simulink model "formula"  (R2019a)
settings: Solver=VariableStepAuto  StartTime=0.0  StopTime=20  RelTol=1e-3
values from neighbouring files (symbols this model uses):
  a0 = 1.3    [mf.mat]    (also in model_2r.m; model_Fy.m)
  a1 = -0.0274    [mf.mat]    (also in model_2r.m; model_Fy.m)
  a10 = 0.015    [mf.mat]    (also in model_2r.m; model_Fy.m)
  a11 = 0.00849    [mf.mat]    (also in model_2r.m = 0.0849; model_Fy.m)
  a12 = -0.0103    [mf.mat]    (also in model_2r.m; model_Fy.m)
  a13 = 0.0395    [mf.mat]    (also in model_2r.m; model_Fy.m)
  a2 = 1.05    [mf.mat]    (also in model_2r.m; model_Fy.m)
  a3 = 1.18    [mf.mat]    (also in model_2r.m; model_Fy.m)
  a4 = 7.69    [mf.mat]    (also in model_2r.m; model_Fy.m)
  a5 = 0.009    [mf.mat]    (also in model_2r.m; model_Fy.m)
  a6 = -0.257    [mf.mat]    (also in model_2r.m; model_Fy.m)
  a7 = 0.224    [mf.mat]    (also in model_2r.m; model_Fy.m)
  a8 = 0.025    [mf.mat]    (also in model_2r.m; model_Fy.m)
  a9 = 0.01    [mf.mat]    (also in model_2r.m; model_Fy.m)
  Iz = 1500    [mf.mat]    (also in model_2r.m)
  lf = 1.4    [mf.mat]    (also in model_2r.m = 1.2)
  lr = 1.2    [mf.mat]    (also in model_2r.m = 1.4)
  m = 1200    [mf.mat]    (also in model_2r.m)
  V = v/3.6    (= 27.7777777778)    [model_2r.m]
settings Model: Creator=Shingo Haketa  LastModifiedBy=hayak

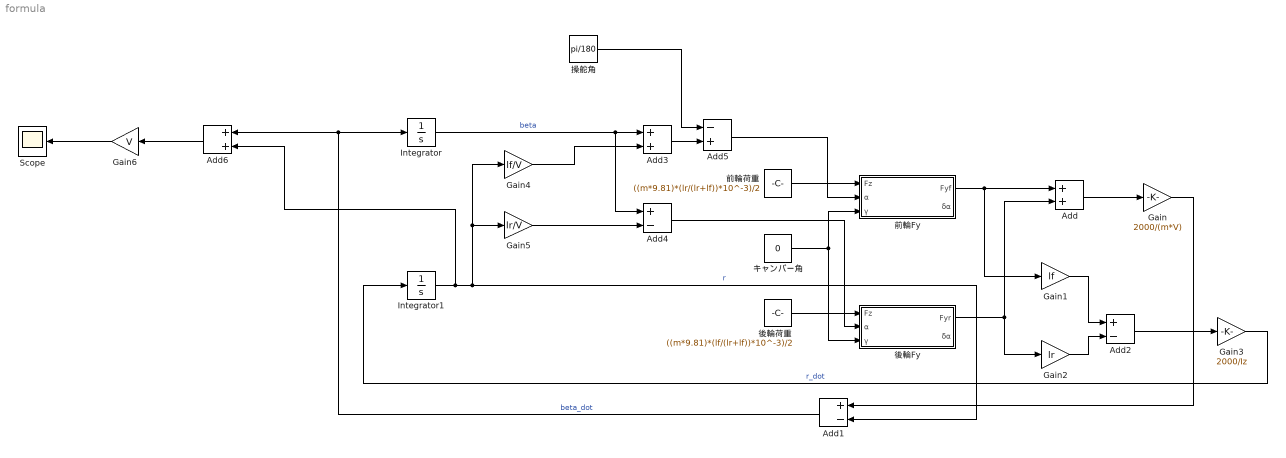
== system formula ==
  Add : Sum
  Add1 : Sum  Inputs=+-
  Add2 : Sum  Inputs=+-
  Add3 : Sum
  Add4 : Sum  Inputs=+-
  Add5 : Sum  Inputs=-+
  Add6 : Sum
  Gain : Gain  Gain=2000/(m*V)
  Gain1 : Gain  Gain=lf
  Gain2 : Gain  Gain=lr
  Gain3 : Gain  Gain=2000/Iz
  Gain4 : Gain  Gain=lf/V
  Gain5 : Gain  Gain=lr/V
  Gain6 : Gain  Gain=V
  Integrator : Integrator
  Integrator1 : Integrator
  Scope : Scope
  キャンバー角 : Constant  Value=0
  前輪Fy : Subsystem
  前輪荷重 : Constant  Value=((m*9.81)*(lr/(lr+lf))*10^-3)/2
  後輪Fy : Subsystem
  後輪荷重 : Constant  Value=((m*9.81)*(lf/(lr+lf))*10^-3)/2
  操舵角 : Constant  Value=pi/180
  wires:
  前輪荷重/1 -> 前輪Fy/1(Fz)
  後輪荷重/1 -> 後輪Fy/1(Fz)
  キャンバー角/1 -> 後輪Fy/3(γ), 前輪Fy/3(γ)
  Integrator/1 -> Add4/1, Add3/1  "beta"
  Add1/1 -> Integrator/1, Add6/1  "beta_dot"
  Integrator1/1 -> Add6/2, Add1/2, Gain5/1, Gain4/1  "r"
  Gain3/1 -> Integrator1/1  "r_dot"
  前輪Fy/1(Fyf) -> Gain1/1, Add/1
  後輪Fy/1(Fyr) -> Gain2/1, Add/2
  Add/1 -> Gain/1
  Gain/1 -> Add1/1
  Gain1/1 -> Add2/1
  Gain2/1 -> Add2/2
  Add2/1 -> Gain3/1
  Gain4/1 -> Add3/2
  操舵角/1 -> Add5/1
  Add3/1 -> Add5/2
  Add5/1 -> 前輪Fy/2(α)
  Gain5/1 -> Add4/2
  Add4/1 -> 後輪Fy/2(α)
  Add6/1 -> Gain6/1
  Gain6/1 -> Scope/1

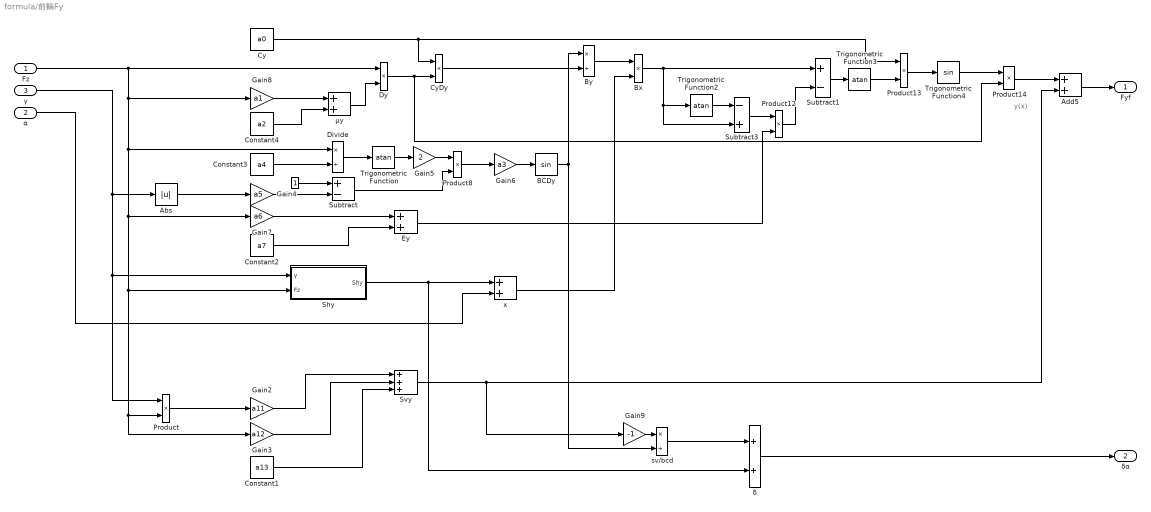
== system formula/前輪Fy ==
  note: y(x)
  Fz : Inport
  α : Inport  Port=2
  γ : Inport  Port=3
  " " : Constant
  Abs : Abs
  Add5 : Sum
  BCDy : Trigonometry
  Bx : Product
  By : Product  Inputs=*/
  Constant1 : Constant  Value=a13
  Constant2 : Constant  Value=a7
  Constant3 : Constant  Value=a4
  Constant4 : Constant  Value=a2
  Cy : Constant  Value=a0
  CyDy : Product
  Divide : Product  Inputs=*/
  Dy : Product
  Ey : Sum
  Gain2 : Gain  Gain=a11
  Gain3 : Gain  Gain=a12
  Gain4 : Gain  Gain=a5
  Gain5 : Gain  Gain=2
  Gain6 : Gain  Gain=a3
  Gain7 : Gain  Gain=a6
  Gain8 : Gain  Gain=a1
  Gain9 : Gain  Gain=-1
  Product{,8,12..14} (5 alike) : Product
  Shy : Subsystem
  Subtract : Sum  Inputs=+-
  Subtract1 : Sum  Inputs=+-
  Subtract3 : Sum  Inputs=-+
  Svy : Sum  Inputs=+++
  Trigonometric Function : Trigonometry  Operator=atan
  Trigonometric Function2 : Trigonometry  Operator=atan
  Trigonometric Function3 : Trigonometry  Operator=atan
  Trigonometric Function4 : Trigonometry
  sv/bcd : Product  Inputs=*/
  x : Sum
  δ : Sum
  μy : Sum
  Fyf : Outport
  δα : Outport  Port=2
  wires:
  Ey/1 -> Product12/2
  γ/1 -> Abs/1, Product/1, Shy/1(γ)
  Product14/1 -> Add5/1
  Trigonometric Function/1 -> Gain5/1
  " "/1 -> Subtract/1
  Gain5/1 -> Product8/1
  Abs/1 -> Gain4/1
  μy/1 -> Dy/2
  Bx/1 -> Subtract3/2, Trigonometric Function2/1, Subtract1/1
  Fz/1 -> Dy/1, Divide/1, Gain7/1, Gain3/1, Product/2, Shy/2(Fz), Gain8/1
  Trigonometric Function3/1 -> Product13/2
  Gain2/1 -> Svy/1
  Product8/1 -> Gain6/1
  Constant3/1 -> Divide/2
  Svy/1 -> Gain9/1, Add5/2
  Gain8/1 -> μy/1
  Gain6/1 -> BCDy/1
  Product12/1 -> Subtract1/2
  Constant1/1 -> Svy/3
  Cy/1 -> CyDy/1, Product13/1
  Subtract/1 -> Product8/2
  Trigonometric Function4/1 -> Product14/1
  Product13/1 -> Trigonometric Function4/1
  CyDy/1 -> By/2
  Dy/1 -> Product14/2, CyDy/2
  Trigonometric Function2/1 -> Subtract3/1
  Constant4/1 -> μy/2
  Gain4/1 -> Subtract/2
  Add5/1 -> Fyf/1
  By/1 -> Bx/1
  BCDy/1 -> By/1, sv/bcd/2
  Subtract3/1 -> Product12/1
  α/1 -> x/2
  Subtract1/1 -> Trigonometric Function3/1
  Shy/1(Shy) -> δ/2, x/1
  Gain3/1 -> Svy/2
  Constant2/1 -> Ey/2
  Product/1 -> Gain2/1
  x/1 -> Bx/2
  Divide/1 -> Trigonometric Function/1
  Gain7/1 -> Ey/1
  Gain9/1 -> sv/bcd/1
  sv/bcd/1 -> δ/1
  δ/1 -> δα/1

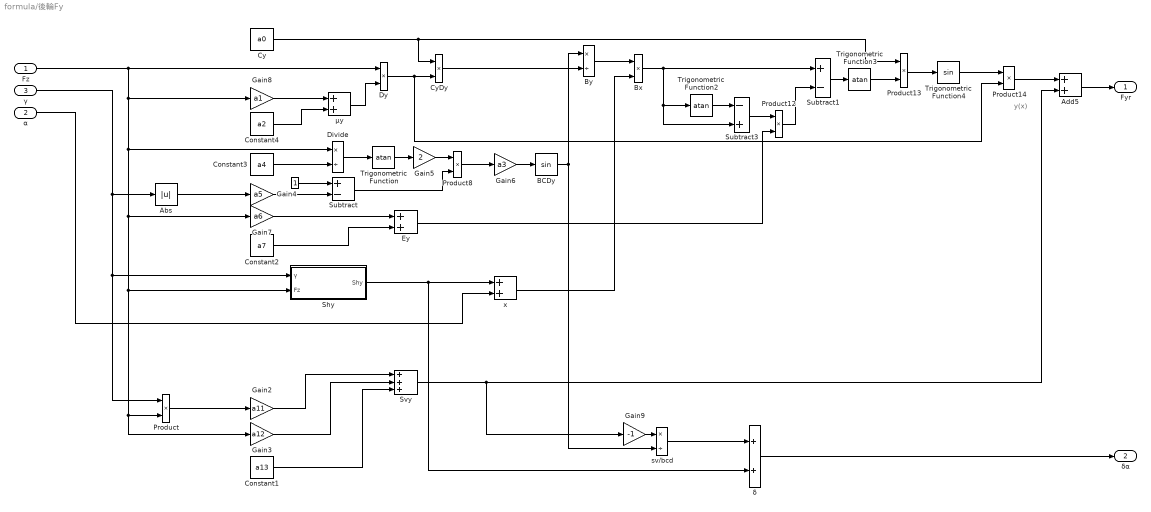
== system formula/後輪Fy ==
  note: y(x)
  Fz : Inport
  α : Inport  Port=2
  γ : Inport  Port=3
  " " : Constant
  Abs : Abs
  Add5 : Sum
  BCDy : Trigonometry
  Bx : Product
  By : Product  Inputs=*/
  Constant1 : Constant  Value=a13
  Constant2 : Constant  Value=a7
  Constant3 : Constant  Value=a4
  Constant4 : Constant  Value=a2
  Cy : Constant  Value=a0
  CyDy : Product
  Divide : Product  Inputs=*/
  Dy : Product
  Ey : Sum
  Gain2 : Gain  Gain=a11
  Gain3 : Gain  Gain=a12
  Gain4 : Gain  Gain=a5
  Gain5 : Gain  Gain=2
  Gain6 : Gain  Gain=a3
  Gain7 : Gain  Gain=a6
  Gain8 : Gain  Gain=a1
  Gain9 : Gain  Gain=-1
  Product{,8,12..14} (5 alike) : Product
  Shy : Subsystem
  Subtract : Sum  Inputs=+-
  Subtract1 : Sum  Inputs=+-
  Subtract3 : Sum  Inputs=-+
  Svy : Sum  Inputs=+++
  Trigonometric Function : Trigonometry  Operator=atan
  Trigonometric Function2 : Trigonometry  Operator=atan
  Trigonometric Function3 : Trigonometry  Operator=atan
  Trigonometric Function4 : Trigonometry
  sv/bcd : Product  Inputs=*/
  x : Sum
  δ : Sum
  μy : Sum
  Fyr : Outport
  δα : Outport  Port=2
  wires:
  Ey/1 -> Product12/2
  γ/1 -> Abs/1, Product/1, Shy/1(γ)
  Product14/1 -> Add5/1
  Trigonometric Function/1 -> Gain5/1
  " "/1 -> Subtract/1
  Gain5/1 -> Product8/1
  Abs/1 -> Gain4/1
  μy/1 -> Dy/2
  Bx/1 -> Subtract3/2, Trigonometric Function2/1, Subtract1/1
  Fz/1 -> Dy/1, Divide/1, Gain7/1, Gain3/1, Product/2, Shy/2(Fz), Gain8/1
  Trigonometric Function3/1 -> Product13/2
  Gain2/1 -> Svy/1
  Product8/1 -> Gain6/1
  Constant3/1 -> Divide/2
  Svy/1 -> Gain9/1, Add5/2
  Gain8/1 -> μy/1
  Gain6/1 -> BCDy/1
  Product12/1 -> Subtract1/2
  Constant1/1 -> Svy/3
  Cy/1 -> CyDy/1, Product13/1
  Subtract/1 -> Product8/2
  Trigonometric Function4/1 -> Product14/1
  Product13/1 -> Trigonometric Function4/1
  CyDy/1 -> By/2
  Dy/1 -> Product14/2, CyDy/2
  Trigonometric Function2/1 -> Subtract3/1
  Constant4/1 -> μy/2
  Gain4/1 -> Subtract/2
  Add5/1 -> Fyr/1
  By/1 -> Bx/1
  BCDy/1 -> By/1, sv/bcd/2
  Subtract3/1 -> Product12/1
  α/1 -> x/2
  Subtract1/1 -> Trigonometric Function3/1
  Shy/1(Shy) -> δ/2, x/1
  Gain3/1 -> Svy/2
  Constant2/1 -> Ey/2
  Product/1 -> Gain2/1
  x/1 -> Bx/2
  Divide/1 -> Trigonometric Function/1
  Gain7/1 -> Ey/1
  Gain9/1 -> sv/bcd/1
  sv/bcd/1 -> δ/1
  δ/1 -> δα/1

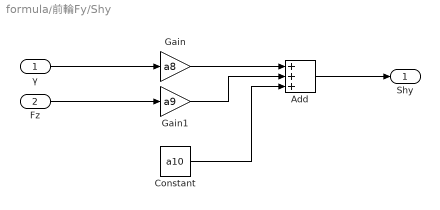
== system formula/前輪Fy/Shy ==
  γ : Inport
  Fz : Inport  Port=2
  Add : Sum  Inputs=+++
  Constant : Constant  Value=a10
  Gain : Gain  Gain=a8
  Gain1 : Gain  Gain=a9
  Shy : Outport  VectorParamsAs1DForOutWhenUnconnected=on
  wires:
  Gain1/1 -> Add/2
  Constant/1 -> Add/3
  Fz/1 -> Gain1/1
  γ/1 -> Gain/1
  Gain/1 -> Add/1
  Add/1 -> Shy/1

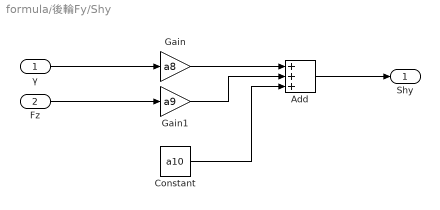
== system formula/後輪Fy/Shy ==
  γ : Inport
  Fz : Inport  Port=2
  Add : Sum  Inputs=+++
  Constant : Constant  Value=a10
  Gain : Gain  Gain=a8
  Gain1 : Gain  Gain=a9
  Shy : Outport  VectorParamsAs1DForOutWhenUnconnected=on
  wires:
  Gain1/1 -> Add/2
  Constant/1 -> Add/3
  Fz/1 -> Gain1/1
  γ/1 -> Gain/1
  Gain/1 -> Add/1
  Add/1 -> Shy/1
